simulink model "hydraulic_model"  (R2024a)
settings: Solver=ode23t  StartTime=0.0  StopTime=tEnd  FixedStep=1e-4  MaxStep=maxStep  RelTol=1e-2  AbsTol=1e-2
values from neighbouring files (symbols this model uses):
  boomHEArea = pi * (boomBoreDiameter/2)^2    (= 3117.24531052)    [init_model.m]
  boomREArea = pi * (boomBoreDiameter/2)^2 - pi*(boomRodDiameter/2)^2    (= 2410.38696347)    [init_model.m]
  swingDisplacement = 23.6    [init_model.m]
undefined symbols (not defined in the file or in its folder): ArmC, ArmR, AToTOrificeVector, BiPOrificeVector, BoomC, BoomR, boomValve, BToTOrificeVector, BucketC, BucketR, bucketValve, fluids, PToAOrificeVector, PToBOrificeVector, stickValve, SwingC, SwingR, swingValve, X, Y, Z
libraries: fl_lib x81, SimscapeFluids_lib x54, sm_lib x34, nesl_utility x29, spsFirstOrderFilterLib x4
(part 2 of 5)

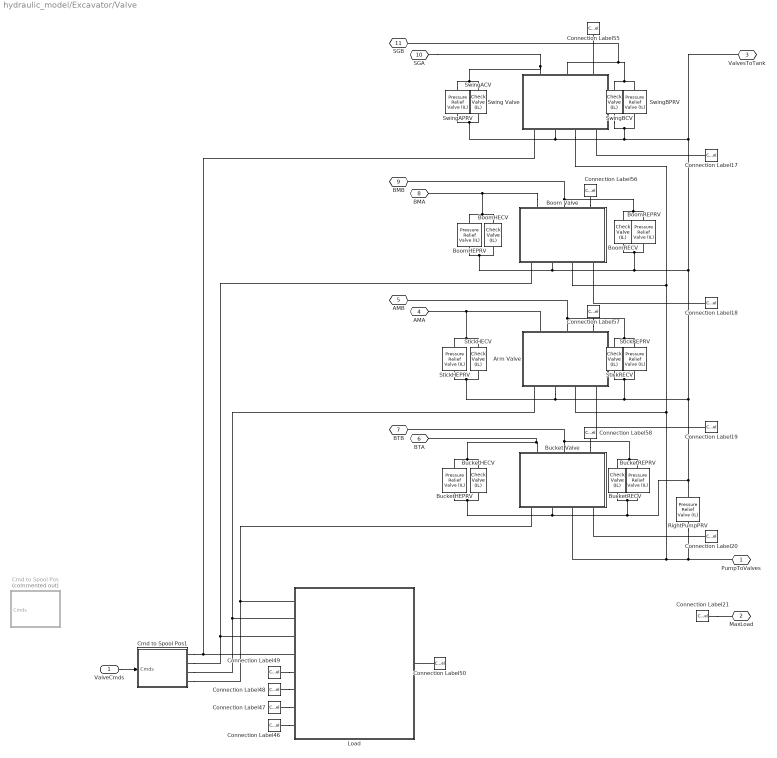
== system hydraulic_model/Excavator/Valve ==
  ValveCmds : Inport
  Arm Valve : Subsystem  mask{valveData=stickValve}
      mask prompts: valveData "Stick Valve Data Structure:"
      mask DialogControl DescGroupVar Prompt: Stick Valve
      mask DialogControl DescTextVar Prompt: The Stick Valve is a 6/3 valve with integrated check valve for induced flow.
      mask Display: image('Valve_6p3w_IMAGE.png');
  Boom Valve : Subsystem  mask{valveData=boomValve}
      mask prompts: valveData "Boom Valve Data Structure:"
      mask DialogControl DescGroupVar Prompt: Boom Valve
      mask DialogControl DescTextVar Prompt: The Boom Valve is a 6/3 valve with integrated check valve for induced flow.
      mask Display: image('Valve_6p3w_IMAGE.png');
  BoomHECV : SimscapeFluids_lib/Isothermal Liquid/Valves & Orifices/Directional Control Valves/Check Valve (IL)  opening_spec=2*(fluids.isothermal_liquid.valves_orifices.enum.opening_spec.linear)-1  pressure_control_spec=fluids.isothermal_liquid.valves_orifices.enum.pressure_control_spec.dp  p_crack_differential=checkValves.crackingPrDiff bar  p_crack_gauge=0.1 MPa  press_max_differential=checkValves.maxOpeningPrDiff bar  press_max_gauge=0.2 MPa  area_max=checkValves.maxOpeningArea mm^2  area_leak=checkValves.leakageArea mm^2  p_diff_TLU=[0.01 : 0.01 : 0.1] MPa  valve_area_TLU=[1e-10, 1e-05, 2e-05, 3e-05, 4e-05, 5e-05, 6e-05, 7.5e-05, 8.5e-05, .0001] m^2  vol_flow_TLU=[.000358, .045, .11, .191, .284, .39, .505, .63, .764, .905] .* 1e-3 m^3/s  area=inf m^2  Cd=0.64  Re_c=150  smoothing_factor=0.01  pressure_recovery=simscape.enum.onoff.off  opening_dynamics=simscape.enum.onoff.off  tau=0.1 s  enable_faults=simscape.enum.onoff.off  fault_action=fluids.enum.FaultOpening.Closed
      settings: InternalSimscapePortConfiguration="{\"Bottom\":[],\"Left\":[{\"id\":\"A\",\"label\":\"A\",\"type\":\"foundation.isothermal_liquid.isothermal_liquid\"}],\"Right\":[{\"id\":\"B\",\"label\":\"B\",\"type\":\"foundation.isothermal_liquid.isothermal_liquid\"}],\"Top\":[]}"
  BoomHEPRV : SimscapeFluids_lib/Isothermal Liquid/Valves & Orifices/Pressure Control Valves/Pressure Relief Valve (IL)  set_pressure_spec=foundation.enum.constant_controlled.constant  opening_spec=fluids.isothermal_liquid.valves_orifices.enum.opening_spec.linear  pressure_spec=fluids.isothermal_liquid.valves_orifices.enum.pressure_control_spec.dp  p_set_gauge=0.1 MPa  p_set_differential=fcnPRV.reliefPr bar  p_range=fcnPRV.regRange bar  area_max=fcnPRV.maxOpeningArea mm^2  area_leak=fcnPRV.leakageArea mm^2  p_diff_TLU=[0.2 : 0.2 : 1.2] MPa  p_gauge_TLU=[0.2 : 0.2 : 1.2] MPa  valve_area_TLU=[1e-10, 2e-06, 4e-06, 6e-06, 8e-06, 1e-05] m^2  vol_flow_TLU=[1e-09, 3.6e-05, 8.9e-05, .00015, .00023, .00031] m^3/s  area=inf m^2  Cd=0.64  Re_c=150  smoothing_factor=0.01  pressure_recovery=simscape.enum.onoff.off  opening_dynamics=simscape.enum.onoff.off  tau=0.1 s  enable_faults=simscape.enum.onoff.off  fault_type=fluids.enum.FaultOpening.Closed
      settings: InternalSimscapePortConfiguration="{\"Bottom\":[],\"Left\":[{\"id\":\"A\",\"label\":\"A\",\"type\":\"foundation.isothermal_liquid.isothermal_liquid\"}],\"Right\":[{\"id\":\"B\",\"label\":\"B\",\"type\":\"foundation.isothermal_liquid.isothermal_liquid\"}],\"Top\":[]}"
  BoomRECV : SimscapeFluids_lib/Isothermal Liquid/Valves & Orifices/Directional Control Valves/Check Valve (IL)  opening_spec=2*(fluids.isothermal_liquid.valves_orifices.enum.opening_spec.linear)-1  pressure_control_spec=fluids.isothermal_liquid.valves_orifices.enum.pressure_control_spec.dp  p_crack_differential=checkValves.crackingPrDiff bar  p_crack_gauge=0.1 MPa  press_max_differential=checkValves.maxOpeningPrDiff bar  press_max_gauge=0.2 MPa  area_max=checkValves.maxOpeningArea mm^2  area_leak=checkValves.leakageArea mm^2  p_diff_TLU=[0.01 : 0.01 : 0.1] MPa  valve_area_TLU=[1e-10, 1e-05, 2e-05, 3e-05, 4e-05, 5e-05, 6e-05, 7.5e-05, 8.5e-05, .0001] m^2  vol_flow_TLU=[.000358, .045, .11, .191, .284, .39, .505, .63, .764, .905] .* 1e-3 m^3/s  area=inf m^2  Cd=0.64  Re_c=150  smoothing_factor=0.01  pressure_recovery=simscape.enum.onoff.off  opening_dynamics=simscape.enum.onoff.off  tau=0.1 s  enable_faults=simscape.enum.onoff.off  fault_action=fluids.enum.FaultOpening.Closed
      settings: InternalSimscapePortConfiguration="{\"Bottom\":[],\"Left\":[{\"id\":\"A\",\"label\":\"A\",\"type\":\"foundation.isothermal_liquid.isothermal_liquid\"}],\"Right\":[{\"id\":\"B\",\"label\":\"B\",\"type\":\"foundation.isothermal_liquid.isothermal_liquid\"}],\"Top\":[]}"
  BoomREPRV : SimscapeFluids_lib/Isothermal Liquid/Valves & Orifices/Pressure Control Valves/Pressure Relief Valve (IL)  set_pressure_spec=foundation.enum.constant_controlled.constant  opening_spec=fluids.isothermal_liquid.valves_orifices.enum.opening_spec.linear  pressure_spec=fluids.isothermal_liquid.valves_orifices.enum.pressure_control_spec.dp  p_set_gauge=0.1 MPa  p_set_differential=fcnPRV.reliefPr bar  p_range=fcnPRV.regRange bar  area_max=fcnPRV.maxOpeningArea mm^2  area_leak=fcnPRV.leakageArea mm^2  p_diff_TLU=[0.2 : 0.2 : 1.2] MPa  p_gauge_TLU=[0.2 : 0.2 : 1.2] MPa  valve_area_TLU=[1e-10, 2e-06, 4e-06, 6e-06, 8e-06, 1e-05] m^2  vol_flow_TLU=[1e-09, 3.6e-05, 8.9e-05, .00015, .00023, .00031] m^3/s  area=inf m^2  Cd=0.64  Re_c=150  smoothing_factor=0.01  pressure_recovery=simscape.enum.onoff.off  opening_dynamics=simscape.enum.onoff.off  tau=0.1 s  enable_faults=simscape.enum.onoff.off  fault_type=fluids.enum.FaultOpening.Closed
      settings: InternalSimscapePortConfiguration="{\"Bottom\":[],\"Left\":[{\"id\":\"A\",\"label\":\"A\",\"type\":\"foundation.isothermal_liquid.isothermal_liquid\"}],\"Right\":[{\"id\":\"B\",\"label\":\"B\",\"type\":\"foundation.isothermal_liquid.isothermal_liquid\"}],\"Top\":[]}"
  Bucket Valve : Subsystem  mask{valveData=bucketValve}
      mask prompts: valveData "Bucket Valve Data Structure:"
      mask DialogControl DescGroupVar Prompt: Bucket Valve
      mask DialogControl DescTextVar Prompt: The Bucket Valve is a 6/3 valve.
      mask Display: image('Valve_6p3w_IMAGE.png');
  BucketHECV : SimscapeFluids_lib/Isothermal Liquid/Valves & Orifices/Directional Control Valves/Check Valve (IL)  opening_spec=2*(fluids.isothermal_liquid.valves_orifices.enum.opening_spec.linear)-1  pressure_control_spec=fluids.isothermal_liquid.valves_orifices.enum.pressure_control_spec.dp  p_crack_differential=checkValves.crackingPrDiff bar  p_crack_gauge=0.1 MPa  press_max_differential=checkValves.maxOpeningPrDiff bar  press_max_gauge=0.2 MPa  area_max=checkValves.maxOpeningArea mm^2  area_leak=checkValves.leakageArea mm^2  p_diff_TLU=[0.01 : 0.01 : 0.1] MPa  valve_area_TLU=[1e-10, 1e-05, 2e-05, 3e-05, 4e-05, 5e-05, 6e-05, 7.5e-05, 8.5e-05, .0001] m^2  vol_flow_TLU=[.000358, .045, .11, .191, .284, .39, .505, .63, .764, .905] .* 1e-3 m^3/s  area=inf m^2  Cd=0.64  Re_c=150  smoothing_factor=0.01  pressure_recovery=simscape.enum.onoff.off  opening_dynamics=simscape.enum.onoff.off  tau=0.1 s  enable_faults=simscape.enum.onoff.off  fault_action=fluids.enum.FaultOpening.Closed
      settings: InternalSimscapePortConfiguration="{\"Bottom\":[],\"Left\":[{\"id\":\"A\",\"label\":\"A\",\"type\":\"foundation.isothermal_liquid.isothermal_liquid\"}],\"Right\":[{\"id\":\"B\",\"label\":\"B\",\"type\":\"foundation.isothermal_liquid.isothermal_liquid\"}],\"Top\":[]}"
  BucketHEPRV : SimscapeFluids_lib/Isothermal Liquid/Valves & Orifices/Pressure Control Valves/Pressure Relief Valve (IL)  set_pressure_spec=foundation.enum.constant_controlled.constant  opening_spec=fluids.isothermal_liquid.valves_orifices.enum.opening_spec.linear  pressure_spec=fluids.isothermal_liquid.valves_orifices.enum.pressure_control_spec.dp  p_set_gauge=0.1 MPa  p_set_differential=fcnPRV.reliefPr bar  p_range=fcnPRV.regRange bar  area_max=fcnPRV.maxOpeningArea mm^2  area_leak=fcnPRV.leakageArea mm^2  p_diff_TLU=[0.2 : 0.2 : 1.2] MPa  p_gauge_TLU=[0.2 : 0.2 : 1.2] MPa  valve_area_TLU=[1e-10, 2e-06, 4e-06, 6e-06, 8e-06, 1e-05] m^2  vol_flow_TLU=[1e-09, 3.6e-05, 8.9e-05, .00015, .00023, .00031] m^3/s  area=inf m^2  Cd=0.64  Re_c=150  smoothing_factor=0.01  pressure_recovery=simscape.enum.onoff.off  opening_dynamics=simscape.enum.onoff.off  tau=0.1 s  enable_faults=simscape.enum.onoff.off  fault_type=fluids.enum.FaultOpening.Closed
      settings: InternalSimscapePortConfiguration="{\"Bottom\":[],\"Left\":[{\"id\":\"A\",\"label\":\"A\",\"type\":\"foundation.isothermal_liquid.isothermal_liquid\"}],\"Right\":[{\"id\":\"B\",\"label\":\"B\",\"type\":\"foundation.isothermal_liquid.isothermal_liquid\"}],\"Top\":[]}"
  BucketRECV : SimscapeFluids_lib/Isothermal Liquid/Valves & Orifices/Directional Control Valves/Check Valve (IL)  opening_spec=2*(fluids.isothermal_liquid.valves_orifices.enum.opening_spec.linear)-1  pressure_control_spec=fluids.isothermal_liquid.valves_orifices.enum.pressure_control_spec.dp  p_crack_differential=checkValves.crackingPrDiff bar  p_crack_gauge=0.1 MPa  press_max_differential=checkValves.maxOpeningPrDiff bar  press_max_gauge=0.2 MPa  area_max=checkValves.maxOpeningArea mm^2  area_leak=checkValves.leakageArea mm^2  p_diff_TLU=[0.01 : 0.01 : 0.1] MPa  valve_area_TLU=[1e-10, 1e-05, 2e-05, 3e-05, 4e-05, 5e-05, 6e-05, 7.5e-05, 8.5e-05, .0001] m^2  vol_flow_TLU=[.000358, .045, .11, .191, .284, .39, .505, .63, .764, .905] .* 1e-3 m^3/s  area=inf m^2  Cd=0.64  Re_c=150  smoothing_factor=0.01  pressure_recovery=simscape.enum.onoff.off  opening_dynamics=simscape.enum.onoff.off  tau=0.1 s  enable_faults=simscape.enum.onoff.off  fault_action=fluids.enum.FaultOpening.Closed
      settings: InternalSimscapePortConfiguration="{\"Bottom\":[],\"Left\":[{\"id\":\"A\",\"label\":\"A\",\"type\":\"foundation.isothermal_liquid.isothermal_liquid\"}],\"Right\":[{\"id\":\"B\",\"label\":\"B\",\"type\":\"foundation.isothermal_liquid.isothermal_liquid\"}],\"Top\":[]}"
  BucketREPRV : SimscapeFluids_lib/Isothermal Liquid/Valves & Orifices/Pressure Control Valves/Pressure Relief Valve (IL)  set_pressure_spec=foundation.enum.constant_controlled.constant  opening_spec=fluids.isothermal_liquid.valves_orifices.enum.opening_spec.linear  pressure_spec=fluids.isothermal_liquid.valves_orifices.enum.pressure_control_spec.dp  p_set_gauge=0.1 MPa  p_set_differential=fcnPRV.reliefPr bar  p_range=fcnPRV.regRange bar  area_max=fcnPRV.maxOpeningArea mm^2  area_leak=fcnPRV.leakageArea mm^2  p_diff_TLU=[0.2 : 0.2 : 1.2] MPa  p_gauge_TLU=[0.2 : 0.2 : 1.2] MPa  valve_area_TLU=[1e-10, 2e-06, 4e-06, 6e-06, 8e-06, 1e-05] m^2  vol_flow_TLU=[1e-09, 3.6e-05, 8.9e-05, .00015, .00023, .00031] m^3/s  area=inf m^2  Cd=0.64  Re_c=150  smoothing_factor=0.01  pressure_recovery=simscape.enum.onoff.off  opening_dynamics=simscape.enum.onoff.off  tau=0.1 s  enable_faults=simscape.enum.onoff.off  fault_type=fluids.enum.FaultOpening.Closed
      settings: InternalSimscapePortConfiguration="{\"Bottom\":[],\"Left\":[{\"id\":\"A\",\"label\":\"A\",\"type\":\"foundation.isothermal_liquid.isothermal_liquid\"}],\"Right\":[{\"id\":\"B\",\"label\":\"B\",\"type\":\"foundation.isothermal_liquid.isothermal_liquid\"}],\"Top\":[]}"
  Cmd to Spool Pos : Subsystem  Commented=on
  Cmd to Spool Pos1 : Subsystem
  Connection Label{17..21,50} (6 alike) : ConnectionLabel  Label=MaxLoad
  Connection Label46 : ConnectionLabel  Label=LoadSG
  Connection Label47 : ConnectionLabel  Label=LoadBM
  Connection Label48 : ConnectionLabel  Label=LoadAM
  Connection Label49 : ConnectionLabel  Label=LoadBT
  Connection Label55 : ConnectionLabel  Label=LoadSG
  Connection Label56 : ConnectionLabel  Label=LoadBM
  Connection Label57 : ConnectionLabel  Label=LoadAM
  Connection Label58 : ConnectionLabel  Label=LoadBT
  Load : Subsystem
  RightPumpPRV : SimscapeFluids_lib/Isothermal Liquid/Valves & Orifices/Pressure Control Valves/Pressure Relief Valve (IL)  set_pressure_spec=foundation.enum.constant_controlled.constant  opening_spec=fluids.isothermal_liquid.valves_orifices.enum.opening_spec.linear  pressure_spec=fluids.isothermal_liquid.valves_orifices.enum.pressure_control_spec.dp  p_set_gauge=0.1 MPa  p_set_differential=pumpPRV.reliefPr bar  p_range=pumpPRV.regRange bar  area_max=pumpPRV.maxOpeningArea mm^2  area_leak=pumpPRV.leakageArea mm^2  p_diff_TLU=[30.15e5 : 15e3 : 31.35e5] Pa  p_gauge_TLU=[30.15e5 : 15e3 : 31.35e5] Pa  valve_area_TLU=[1 : 1 : 9] .* 1e-5 m^2  vol_flow_TLU=[1e-09, 3.6e-05, 8.9e-05, .00015, .00023, .00031] m^3/s  area=inf m^2  Cd=0.64  Re_c=150  smoothing_factor=0.1  pressure_recovery=simscape.enum.onoff.off  opening_dynamics=simscape.enum.onoff.off  tau=0.1 s  enable_faults=simscape.enum.onoff.off  fault_type=fluids.enum.FaultOpening.Closed
      settings: InternalSimscapePortConfiguration="{\"Bottom\":[],\"Left\":[{\"id\":\"A\",\"label\":\"A\",\"type\":\"foundation.isothermal_liquid.isothermal_liquid\"}],\"Right\":[{\"id\":\"B\",\"label\":\"B\",\"type\":\"foundation.isothermal_liquid.isothermal_liquid\"}],\"Top\":[]}"
  StickHECV : SimscapeFluids_lib/Isothermal Liquid/Valves & Orifices/Directional Control Valves/Check Valve (IL)  opening_spec=2*(fluids.isothermal_liquid.valves_orifices.enum.opening_spec.linear)-1  pressure_control_spec=fluids.isothermal_liquid.valves_orifices.enum.pressure_control_spec.dp  p_crack_differential=checkValves.crackingPrDiff bar  p_crack_gauge=0.1 MPa  press_max_differential=checkValves.maxOpeningPrDiff bar  press_max_gauge=0.2 MPa  area_max=checkValves.maxOpeningArea mm^2  area_leak=checkValves.leakageArea mm^2  p_diff_TLU=[0.01 : 0.01 : 0.1] MPa  valve_area_TLU=[1e-10, 1e-05, 2e-05, 3e-05, 4e-05, 5e-05, 6e-05, 7.5e-05, 8.5e-05, .0001] m^2  vol_flow_TLU=[.000358, .045, .11, .191, .284, .39, .505, .63, .764, .905] .* 1e-3 m^3/s  area=inf m^2  Cd=0.64  Re_c=150  smoothing_factor=0.01  pressure_recovery=simscape.enum.onoff.off  opening_dynamics=simscape.enum.onoff.off  tau=0.1 s  enable_faults=simscape.enum.onoff.off  fault_action=fluids.enum.FaultOpening.Closed
      settings: InternalSimscapePortConfiguration="{\"Bottom\":[],\"Left\":[{\"id\":\"A\",\"label\":\"A\",\"type\":\"foundation.isothermal_liquid.isothermal_liquid\"}],\"Right\":[{\"id\":\"B\",\"label\":\"B\",\"type\":\"foundation.isothermal_liquid.isothermal_liquid\"}],\"Top\":[]}"
  StickHEPRV : SimscapeFluids_lib/Isothermal Liquid/Valves & Orifices/Pressure Control Valves/Pressure Relief Valve (IL)  set_pressure_spec=foundation.enum.constant_controlled.constant  opening_spec=fluids.isothermal_liquid.valves_orifices.enum.opening_spec.linear  pressure_spec=fluids.isothermal_liquid.valves_orifices.enum.pressure_control_spec.dp  p_set_gauge=0.1 MPa  p_set_differential=fcnPRV.reliefPr bar  p_range=fcnPRV.regRange bar  area_max=fcnPRV.maxOpeningArea mm^2  area_leak=fcnPRV.leakageArea mm^2  p_diff_TLU=[0.2 : 0.2 : 1.2] MPa  p_gauge_TLU=[0.2 : 0.2 : 1.2] MPa  valve_area_TLU=[1e-10, 2e-06, 4e-06, 6e-06, 8e-06, 1e-05] m^2  vol_flow_TLU=[1e-09, 3.6e-05, 8.9e-05, .00015, .00023, .00031] m^3/s  area=inf m^2  Cd=0.64  Re_c=150  smoothing_factor=0.01  pressure_recovery=simscape.enum.onoff.off  opening_dynamics=simscape.enum.onoff.off  tau=0.1 s  enable_faults=simscape.enum.onoff.off  fault_type=fluids.enum.FaultOpening.Closed
      settings: InternalSimscapePortConfiguration="{\"Bottom\":[],\"Left\":[{\"id\":\"A\",\"label\":\"A\",\"type\":\"foundation.isothermal_liquid.isothermal_liquid\"}],\"Right\":[{\"id\":\"B\",\"label\":\"B\",\"type\":\"foundation.isothermal_liquid.isothermal_liquid\"}],\"Top\":[]}"
  StickRECV : SimscapeFluids_lib/Isothermal Liquid/Valves & Orifices/Directional Control Valves/Check Valve (IL)  opening_spec=2*(fluids.isothermal_liquid.valves_orifices.enum.opening_spec.linear)-1  pressure_control_spec=fluids.isothermal_liquid.valves_orifices.enum.pressure_control_spec.dp  p_crack_differential=checkValves.crackingPrDiff bar  p_crack_gauge=0.1 MPa  press_max_differential=checkValves.maxOpeningPrDiff bar  press_max_gauge=0.2 MPa  area_max=checkValves.maxOpeningArea mm^2  area_leak=checkValves.leakageArea mm^2  p_diff_TLU=[0.01 : 0.01 : 0.1] MPa  valve_area_TLU=[1e-10, 1e-05, 2e-05, 3e-05, 4e-05, 5e-05, 6e-05, 7.5e-05, 8.5e-05, .0001] m^2  vol_flow_TLU=[.000358, .045, .11, .191, .284, .39, .505, .63, .764, .905] .* 1e-3 m^3/s  area=inf m^2  Cd=0.64  Re_c=150  smoothing_factor=0.01  pressure_recovery=simscape.enum.onoff.off  opening_dynamics=simscape.enum.onoff.off  tau=0.1 s  enable_faults=simscape.enum.onoff.off  fault_action=fluids.enum.FaultOpening.Closed
      settings: InternalSimscapePortConfiguration="{\"Bottom\":[],\"Left\":[{\"id\":\"A\",\"label\":\"A\",\"type\":\"foundation.isothermal_liquid.isothermal_liquid\"}],\"Right\":[{\"id\":\"B\",\"label\":\"B\",\"type\":\"foundation.isothermal_liquid.isothermal_liquid\"}],\"Top\":[]}"
  StickREPRV : SimscapeFluids_lib/Isothermal Liquid/Valves & Orifices/Pressure Control Valves/Pressure Relief Valve (IL)  set_pressure_spec=foundation.enum.constant_controlled.constant  opening_spec=fluids.isothermal_liquid.valves_orifices.enum.opening_spec.linear  pressure_spec=fluids.isothermal_liquid.valves_orifices.enum.pressure_control_spec.dp  p_set_gauge=0.1 MPa  p_set_differential=fcnPRV.reliefPr bar  p_range=fcnPRV.regRange bar  area_max=fcnPRV.maxOpeningArea mm^2  area_leak=fcnPRV.leakageArea mm^2  p_diff_TLU=[0.2 : 0.2 : 1.2] MPa  p_gauge_TLU=[0.2 : 0.2 : 1.2] MPa  valve_area_TLU=[1e-10, 2e-06, 4e-06, 6e-06, 8e-06, 1e-05] m^2  vol_flow_TLU=[1e-09, 3.6e-05, 8.9e-05, .00015, .00023, .00031] m^3/s  area=inf m^2  Cd=0.64  Re_c=150  smoothing_factor=0.01  pressure_recovery=simscape.enum.onoff.off  opening_dynamics=simscape.enum.onoff.off  tau=0.1 s  enable_faults=simscape.enum.onoff.off  fault_type=fluids.enum.FaultOpening.Closed
      settings: InternalSimscapePortConfiguration="{\"Bottom\":[],\"Left\":[{\"id\":\"A\",\"label\":\"A\",\"type\":\"foundation.isothermal_liquid.isothermal_liquid\"}],\"Right\":[{\"id\":\"B\",\"label\":\"B\",\"type\":\"foundation.isothermal_liquid.isothermal_liquid\"}],\"Top\":[]}"
  Swing Valve : Subsystem  mask{valveData=swingValve}
      mask prompts: valveData "Swing Valve Data Structure:"
      mask DialogControl DescGroupVar Prompt: Swing Valve
      mask DialogControl DescTextVar Prompt: The Swing Valve is a 6/3 valve.
      mask Display: image('Valve_6p3w_IMAGE.png');
  SwingACV : SimscapeFluids_lib/Isothermal Liquid/Valves & Orifices/Directional Control Valves/Check Valve (IL)  opening_spec=2*(fluids.isothermal_liquid.valves_orifices.enum.opening_spec.linear)-1  pressure_control_spec=fluids.isothermal_liquid.valves_orifices.enum.pressure_control_spec.dp  p_crack_differential=checkValves.crackingPrDiff bar  p_crack_gauge=0.1 MPa  press_max_differential=checkValves.maxOpeningPrDiff bar  press_max_gauge=0.2 MPa  area_max=checkValves.maxOpeningArea mm^2  area_leak=checkValves.leakageArea mm^2  p_diff_TLU=[0.01 : 0.01 : 0.1] MPa  valve_area_TLU=[1e-10, 1e-05, 2e-05, 3e-05, 4e-05, 5e-05, 6e-05, 7.5e-05, 8.5e-05, .0001] m^2  vol_flow_TLU=[.000358, .045, .11, .191, .284, .39, .505, .63, .764, .905] .* 1e-3 m^3/s  area=inf m^2  Cd=0.64  Re_c=150  smoothing_factor=0.01  pressure_recovery=simscape.enum.onoff.off  opening_dynamics=simscape.enum.onoff.off  tau=0.1 s  enable_faults=simscape.enum.onoff.off  fault_action=fluids.enum.FaultOpening.Closed
      settings: InternalSimscapePortConfiguration="{\"Bottom\":[],\"Left\":[{\"id\":\"A\",\"label\":\"A\",\"type\":\"foundation.isothermal_liquid.isothermal_liquid\"}],\"Right\":[{\"id\":\"B\",\"label\":\"B\",\"type\":\"foundation.isothermal_liquid.isothermal_liquid\"}],\"Top\":[]}"
  SwingAPRV : SimscapeFluids_lib/Isothermal Liquid/Valves & Orifices/Pressure Control Valves/Pressure Relief Valve (IL)  set_pressure_spec=foundation.enum.constant_controlled.constant  opening_spec=fluids.isothermal_liquid.valves_orifices.enum.opening_spec.linear  pressure_spec=fluids.isothermal_liquid.valves_orifices.enum.pressure_control_spec.dp  p_set_gauge=0.1 MPa  p_set_differential=swingPRV.reliefPr bar  p_range=swingPRV.regRange bar  area_max=swingPRV.maxOpeningArea mm^2  area_leak=swingPRV.leakageArea mm^2  p_diff_TLU=[0.2 : 0.2 : 1.2] MPa  p_gauge_TLU=[0.2 : 0.2 : 1.2] MPa  valve_area_TLU=[1e-10, 2e-06, 4e-06, 6e-06, 8e-06, 1e-05] m^2  vol_flow_TLU=[1e-09, 3.6e-05, 8.9e-05, .00015, .00023, .00031] m^3/s  area=inf m^2  Cd=0.64  Re_c=150  smoothing_factor=0.01  pressure_recovery=simscape.enum.onoff.off  opening_dynamics=simscape.enum.onoff.off  tau=0.1 s  enable_faults=simscape.enum.onoff.off  fault_type=fluids.enum.FaultOpening.Closed
      settings: InternalSimscapePortConfiguration="{\"Bottom\":[],\"Left\":[{\"id\":\"A\",\"label\":\"A\",\"type\":\"foundation.isothermal_liquid.isothermal_liquid\"}],\"Right\":[{\"id\":\"B\",\"label\":\"B\",\"type\":\"foundation.isothermal_liquid.isothermal_liquid\"}],\"Top\":[]}"
  SwingBCV : SimscapeFluids_lib/Isothermal Liquid/Valves & Orifices/Directional Control Valves/Check Valve (IL)  opening_spec=2*(fluids.isothermal_liquid.valves_orifices.enum.opening_spec.linear)-1  pressure_control_spec=fluids.isothermal_liquid.valves_orifices.enum.pressure_control_spec.dp  p_crack_differential=checkValves.crackingPrDiff bar  p_crack_gauge=0.1 MPa  press_max_differential=checkValves.maxOpeningPrDiff bar  press_max_gauge=0.2 MPa  area_max=checkValves.maxOpeningArea mm^2  area_leak=checkValves.leakageArea mm^2  p_diff_TLU=[0.01 : 0.01 : 0.1] MPa  valve_area_TLU=[1e-10, 1e-05, 2e-05, 3e-05, 4e-05, 5e-05, 6e-05, 7.5e-05, 8.5e-05, .0001] m^2  vol_flow_TLU=[.000358, .045, .11, .191, .284, .39, .505, .63, .764, .905] .* 1e-3 m^3/s  area=inf m^2  Cd=0.64  Re_c=150  smoothing_factor=0.01  pressure_recovery=simscape.enum.onoff.off  opening_dynamics=simscape.enum.onoff.off  tau=0.1 s  enable_faults=simscape.enum.onoff.off  fault_action=fluids.enum.FaultOpening.Closed
      settings: InternalSimscapePortConfiguration="{\"Bottom\":[],\"Left\":[{\"id\":\"A\",\"label\":\"A\",\"type\":\"foundation.isothermal_liquid.isothermal_liquid\"}],\"Right\":[{\"id\":\"B\",\"label\":\"B\",\"type\":\"foundation.isothermal_liquid.isothermal_liquid\"}],\"Top\":[]}"
  SwingBPRV : SimscapeFluids_lib/Isothermal Liquid/Valves & Orifices/Pressure Control Valves/Pressure Relief Valve (IL)  set_pressure_spec=foundation.enum.constant_controlled.constant  opening_spec=fluids.isothermal_liquid.valves_orifices.enum.opening_spec.linear  pressure_spec=fluids.isothermal_liquid.valves_orifices.enum.pressure_control_spec.dp  p_set_gauge=0.1 MPa  p_set_differential=swingPRV.reliefPr bar  p_range=swingPRV.regRange bar  area_max=swingPRV.maxOpeningArea mm^2  area_leak=swingPRV.leakageArea mm^2  p_diff_TLU=[0.2 : 0.2 : 1.2] MPa  p_gauge_TLU=[0.2 : 0.2 : 1.2] MPa  valve_area_TLU=[1e-10, 2e-06, 4e-06, 6e-06, 8e-06, 1e-05] m^2  vol_flow_TLU=[1e-09, 3.6e-05, 8.9e-05, .00015, .00023, .00031] m^3/s  area=inf m^2  Cd=0.64  Re_c=150  smoothing_factor=0.01  pressure_recovery=simscape.enum.onoff.off  opening_dynamics=simscape.enum.onoff.off  tau=0.1 s  enable_faults=simscape.enum.onoff.off  fault_type=fluids.enum.FaultOpening.Closed
      settings: InternalSimscapePortConfiguration="{\"Bottom\":[],\"Left\":[{\"id\":\"A\",\"label\":\"A\",\"type\":\"foundation.isothermal_liquid.isothermal_liquid\"}],\"Right\":[{\"id\":\"B\",\"label\":\"B\",\"type\":\"foundation.isothermal_liquid.isothermal_liquid\"}],\"Top\":[]}"
  PumpToValves : PMIOPort  Side=Left
  MaxLoad : PMIOPort  Port=2  Side=Left
  ValvesToTank : PMIOPort  Port=3  Side=Left
  AMA : PMIOPort  Port=4  Side=Right
  AMB : PMIOPort  Port=5  Side=Right
  BTA : PMIOPort  Port=6  Side=Right
  BTB : PMIOPort  Port=7  Side=Right
  BMA : PMIOPort  Port=8  Side=Right
  BMB : PMIOPort  Port=9  Side=Right
  SGA : PMIOPort  Port=10  Side=Right
  SGB : PMIOPort  Port=11  Side=Right
  wires:
  ValveCmds/1 -> Cmd to Spool Pos1/1(Cmds)
  connections:
  AMA/RConn1 -- StickHECV/RConn1 -- StickHEPRV/LConn1 -- Arm Valve/RConn1
  SwingBPRV/LConn1 -- SwingBCV/RConn1 -- SGB/RConn1 -- Swing Valve/RConn2
  BTA/RConn1 -- Bucket Valve/RConn1 -- BucketHECV/RConn1 -- BucketHEPRV/LConn1
  Bucket Valve/RConn2 -- BucketRECV/RConn1 -- BucketREPRV/LConn1 -- BTB/RConn1
  StickREPRV/LConn1 -- StickRECV/RConn1 -- Arm Valve/RConn2 -- AMB/RConn1
  SwingAPRV/LConn1 -- SGA/RConn1 -- Swing Valve/RConn1 -- SwingACV/RConn1
  Connection Label17/LConn1 -- Swing Valve/LConn4
  Connection Label19/LConn1 -- Arm Valve/LConn4
  Connection Label20/LConn1 -- Bucket Valve/LConn4
  Connection Label21/LConn1 -- MaxLoad/RConn1
  Connection Label18/LConn1 -- Boom Valve/LConn4
  SwingBPRV/RConn1 -- Swing Valve/LConn2 -- SwingACV/LConn1 -- SwingAPRV/RConn1 -- ValvesToTank/RConn1 -- BucketHEPRV/RConn1 -- BucketHECV/LConn1 -- Bucket Valve/LConn2 -- BucketREPRV/RConn1 -- BucketRECV/LConn1 -- RightPumpPRV/RConn1 -- StickHECV/LConn1 -- StickHEPRV/RConn1 -- Arm Valve/LConn2 -- StickRECV/LConn1 -- StickREPRV/RConn1 -- BoomHEPRV/RConn1 -- BoomHECV/LConn1 -- Boom Valve/LConn2 -- BoomRECV/LConn1 -- BoomREPRV/RConn1 -- SwingBCV/LConn1
  Swing Valve/LConn3 -- Boom Valve/LConn3 -- Arm Valve/LConn3 -- Bucket Valve/LConn3 -- PumpToValves/RConn1 -- RightPumpPRV/LConn1
  Connection Label55/LConn1 -- Swing Valve/RConn3
  Connection Label56/LConn1 -- Boom Valve/RConn3
  Connection Label57/LConn1 -- Arm Valve/RConn3
  Connection Label58/LConn1 -- Bucket Valve/RConn3
  Connection Label46/LConn1 -- Load/LConn8
  Connection Label47/LConn1 -- Load/LConn7
  Connection Label48/LConn1 -- Load/LConn6
  Connection Label49/LConn1 -- Load/LConn5
  Connection Label50/LConn1 -- Load/RConn1
  Boom Valve/RConn2 -- BoomREPRV/LConn1 -- BoomRECV/RConn1 -- BMB/RConn1
  Boom Valve/RConn1 -- BMA/RConn1 -- BoomHEPRV/LConn1 -- BoomHECV/RConn1
  Cmd to Spool Pos1/RConn1 -- Load/LConn4 -- Swing Valve/LConn1
  Cmd to Spool Pos1/RConn2 -- Load/LConn3 -- Boom Valve/LConn1
  Cmd to Spool Pos1/RConn3 -- Load/LConn2 -- Arm Valve/LConn1
  Cmd to Spool Pos1/RConn4 -- Load/LConn1 -- Bucket Valve/LConn1

== system hydraulic_model/Excavator/Functions/Arm ==
  ArmCylinder : SimscapeFluids_lib/Isothermal Liquid/Actuators/Double-Acting Actuator (IL)  single_fluid=true  mech_orientation=foundation.enum.MechOrientationTranslational.Positive  piston_area_A=stickHEArea mm^2  piston_area_B=stickREArea mm^2  stroke=stickStroke mm  dead_volume_A=1e-3 m^3  dead_volume_B=1e-3 m^3  pressure_spec=foundation.enum.pressure_spec.atmospheric  environment_pressure=0.101325 MPa  hardstop_model=simscape.enum.hardstop.smooth  stiff_coeff=1e8 N/m  damping_coeff=1e5 N/(m/s)  transition=0.1 mm  coeff_rest=0.7  v_tol=0.001 m/s  f_tol=0.001 N  cushion_A_spec=simscape.enum.onoff.off  area_plunger_A=1e-4 m^2  length_plunger_A=1e-3 m  area_cushion_orifice_A=1e-6 m^2  area_leak_plunger_A=1e-7 m^2  p_crack_differential_A=0.01 MPa  press_max_differential_A=0.1 MPa  check_valve_area_max_A=1e-4 m^2  check_valve_area_leak_A=1e-10 m^2  smoothing_factor_A=0  cushion_B_spec=simscape.enum.onoff.off  area_plunger_B=1e-4 m^2  length_plunger_B=1e-3 m  area_cushion_orifice_B=1e-6 m^2  area_leak_plunger_B=1e-7 m^2  p_crack_differential_B=0.01 MPa  press_max_differential_B=0.1 MPa  check_valve_area_max_B=1e-4 m^2  check_valve_area_leak_B=1e-10 m^2  smoothing_factor_B=0  friction_spec=true  breakaway_Coulomb_ratio=stickCylFriction.brkawyToCoulRatio  breakaway_velocity=stickCylFriction.brkawyVel m/s  preload_force=stickCylFriction.preloadForce N  Coulomb_coeff=stickCylFriction.coulForceCoef N/Pa  viscous_coeff=stickCylFriction.viscCoeff N/(m/s)  leakage_spec=simscape.enum.onoff.off  clearance=1e-4 m  piston_length=0.01 m  displacement_spec=foundation.enum.DisplacementSpec.Calculate  x0=initStickPistonPos m  dynamic_compressibility=simscape.enum.onoff.on  p0_A=initStickHEPr bar  p0_B=initStickREPr bar
      settings: InternalSimscapePortConfiguration="{\"Bottom\":[],\"Left\":[{\"id\":\"C\",\"label\":\"C\",\"type\":\"foundation.mechanical.translational.translational\"},{\"id\":\"A\",\"label\":\"A\",\"type\":\"foundation.isothermal_liquid.isothermal_liquid\"}],\"Right\":[{\"id\":\"p_out\",\"label\":\"p\",\"type\":\"output\"},{\"id\":\"R\",\"label\":\"R\",\"type\":\"foundation.mechanical.translational.translational\"},{\"id\":\"B\",\"label\":\"B\",\"type\":\"foundation.isothermal_liquid.isothermal_liquid\"}],\"Top\":[]}"
  BoomTranslationalRef1 : fl_lib/Mechanical/Translational Elements/Mechanical Translational Reference
  Ideal Translational Motion Sensor : fl_lib/Mechanical/Mechanical Sensors/Ideal Translational Motion Sensor  reference=foundation.enum.MeasurementReference.difference  acceleration_port=false  velocity_port=true  position_port=true  offset=armBias m
  PS Terminator : fl_lib/Physical Signals/Sinks/PS Terminator
  PS-Simulink Converter3 : nesl_utility/PS-Simulink Converter  PhysicalDomain=network_engine_domain  SubClassName=ps_output  LeftPortType=input  RightPortType=output  PseudoPeriodic=off  Frequencies=[]  VectorFormat=1-D array  Unit=m  AffineConversion=off
  PS-Simulink Converter5 : nesl_utility/PS-Simulink Converter  PhysicalDomain=network_engine_domain  SubClassName=ps_output  LeftPortType=input  RightPortType=output  PseudoPeriodic=off  Frequencies=[]  VectorFormat=1-D array  Unit=m/s  AffineConversion=off
  Simscape Bus : SimscapeBus  HierarchyStrings=ArmC;ArmR
  StickTranslationalRef : fl_lib/Mechanical/Translational Elements/Mechanical Translational Reference
  To Workspace : ToWorkspace  VariableName=posArm  SampleTime=-1
      settings: Save2DSignal=2-D array (concatenate along first dimension)
  To Workspace2 : ToWorkspace  VariableName=velArm  SampleTime=-1
      settings: Save2DSignal=2-D array (concatenate along first dimension)
  ArmA : PMIOPort  Side=Left
  ArmB : PMIOPort  Port=2  Side=Left
  ArmHydToMech : PMIOPort  Port=3  Side=Right
  wires:
  PS-Simulink Converter5/1 -> To Workspace2/1
  PS-Simulink Converter3/1 -> To Workspace/1
  connections:
  Ideal Translational Motion Sensor/LConn1 -- ArmCylinder/RConn2 -- Simscape Bus/LConn2
  ArmCylinder/RConn3 -- ArmB/RConn1
  ArmCylinder/LConn2 -- ArmA/RConn1
  ArmCylinder/LConn1 -- Simscape Bus/LConn1 -- StickTranslationalRef/LConn1
  BoomTranslationalRef1/LConn1 -- Ideal Translational Motion Sensor/RConn1
  PS-Simulink Converter3/LConn1 -- Ideal Translational Motion Sensor/RConn3
  Simscape Bus/RConn1 -- ArmHydToMech/RConn1
  PS-Simulink Converter5/LConn1 -- Ideal Translational Motion Sensor/RConn2
  ArmCylinder/RConn1 -- PS Terminator/LConn1

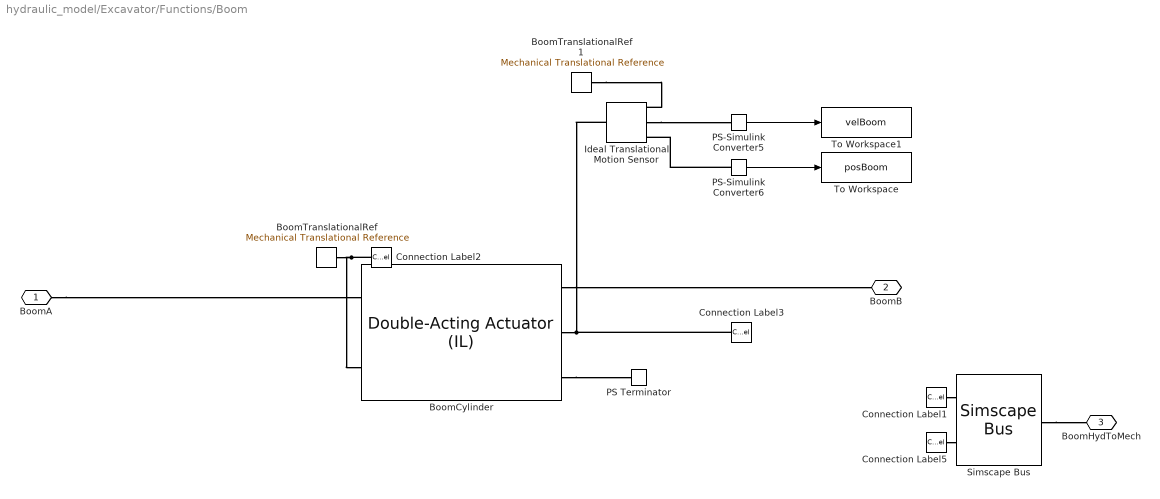
== system hydraulic_model/Excavator/Functions/Boom ==
  BoomCylinder : SimscapeFluids_lib/Isothermal Liquid/Actuators/Double-Acting Actuator (IL)  single_fluid=true  mech_orientation=foundation.enum.MechOrientationTranslational.Positive  piston_area_A=boomHEArea mm^2  piston_area_B=boomREArea mm^2  stroke=boomStroke mm  dead_volume_A=1e-4 m^3  dead_volume_B=1e-4 m^3  pressure_spec=foundation.enum.pressure_spec.atmospheric  environment_pressure=0.101325 MPa  hardstop_model=simscape.enum.hardstop.smooth  stiff_coeff=1e8 N/m  damping_coeff=1e5 N/(m/s)  transition=0.1 mm  coeff_rest=0.7  v_tol=0.001 m/s  f_tol=0.001 N  cushion_A_spec=false  area_plunger_A=boomHEArea/3 mm^2  length_plunger_A=5 mm  area_cushion_orifice_A=5 mm^2  area_leak_plunger_A=1e-7 m^2  p_crack_differential_A=0.01 MPa  press_max_differential_A=0.1 MPa  check_valve_area_max_A=1e-4 m^2  check_valve_area_leak_A=1e-10 m^2  smoothing_factor_A=0  cushion_B_spec=false  area_plunger_B=boomREArea/3 mm^2  length_plunger_B=5 mm  area_cushion_orifice_B=5 mm^2  area_leak_plunger_B=1e-7 m^2  p_crack_differential_B=0.01 MPa  press_max_differential_B=0.1 MPa  check_valve_area_max_B=1e-4 m^2  check_valve_area_leak_B=1e-10 m^2  smoothing_factor_B=0  friction_spec=true  breakaway_Coulomb_ratio=boomCylFriction.brkawyToCoulRatio  breakaway_velocity=boomCylFriction.brkawyVel m/s  preload_force=boomCylFriction.preloadForce N  Coulomb_coeff=boomCylFriction.coulForceCoef N/Pa  viscous_coeff=boomCylFriction.viscCoeff N/(m/s)  leakage_spec=simscape.enum.onoff.off  clearance=1e-4 m  piston_length=0.01 m  displacement_spec=foundation.enum.DisplacementSpec.Calculate  x0=initBoomPistonPos m  dynamic_compressibility=simscape.enum.onoff.on  p0_A=initBoomHEPr bar  p0_B=initBoomREPr bar
      settings: InternalSimscapePortConfiguration="{\"Bottom\":[],\"Left\":[{\"id\":\"C\",\"label\":\"C\",\"type\":\"foundation.mechanical.translational.translational\"},{\"id\":\"A\",\"label\":\"A\",\"type\":\"foundation.isothermal_liquid.isothermal_liquid\"}],\"Right\":[{\"id\":\"p_out\",\"label\":\"p\",\"type\":\"output\"},{\"id\":\"R\",\"label\":\"R\",\"type\":\"foundation.mechanical.translational.translational\"},{\"id\":\"B\",\"label\":\"B\",\"type\":\"foundation.isothermal_liquid.isothermal_liquid\"}],\"Top\":[]}"
  BoomTranslationalRef : fl_lib/Mechanical/Translational Elements/Mechanical Translational Reference
  BoomTranslationalRef1 : fl_lib/Mechanical/Translational Elements/Mechanical Translational Reference
  Connection Label1 : ConnectionLabel  Label=C
  Connection Label2 : ConnectionLabel  Label=C
  Connection Label3 : ConnectionLabel  Label=R
  Connection Label5 : ConnectionLabel  Label=R
  Ideal Translational Motion Sensor : fl_lib/Mechanical/Mechanical Sensors/Ideal Translational Motion Sensor  reference=foundation.enum.MeasurementReference.difference  acceleration_port=false  velocity_port=true  position_port=true  offset=boomBias m
  PS Terminator : fl_lib/Physical Signals/Sinks/PS Terminator
  PS-Simulink Converter5 : nesl_utility/PS-Simulink Converter  PhysicalDomain=network_engine_domain  SubClassName=ps_output  LeftPortType=input  RightPortType=output  PseudoPeriodic=off  Frequencies=[]  VectorFormat=1-D array  Unit=m/s  AffineConversion=off
  PS-Simulink Converter6 : nesl_utility/PS-Simulink Converter  PhysicalDomain=network_engine_domain  SubClassName=ps_output  LeftPortType=input  RightPortType=output  PseudoPeriodic=off  Frequencies=[]  VectorFormat=1-D array  Unit=m  AffineConversion=off
  Simscape Bus : SimscapeBus  HierarchyStrings=BoomC;BoomR
  To Workspace : ToWorkspace  VariableName=posBoom  SampleTime=-1
      settings: Save2DSignal=2-D array (concatenate along first dimension)
  To Workspace1 : ToWorkspace  VariableName=velBoom  SampleTime=-1
      settings: Save2DSignal=2-D array (concatenate along first dimension)
  BoomA : PMIOPort  Side=Left
  BoomB : PMIOPort  Port=2  Side=Left
  BoomHydToMech : PMIOPort  Port=3  Side=Right
  wires:
  PS-Simulink Converter5/1 -> To Workspace1/1
  PS-Simulink Converter6/1 -> To Workspace/1
  connections:
  BoomTranslationalRef/LConn1 -- BoomCylinder/LConn1 -- Connection Label2/LConn1
  BoomA/RConn1 -- BoomCylinder/LConn2
  BoomCylinder/RConn2 -- Connection Label3/LConn1 -- Ideal Translational Motion Sensor/LConn1
  BoomCylinder/RConn3 -- BoomB/RConn1
  BoomTranslationalRef1/LConn1 -- Ideal Translational Motion Sensor/RConn1
  Ideal Translational Motion Sensor/RConn2 -- PS-Simulink Converter5/LConn1
  PS-Simulink Converter6/LConn1 -- Ideal Translational Motion Sensor/RConn3
  Connection Label1/LConn1 -- Simscape Bus/LConn1
  Simscape Bus/RConn1 -- BoomHydToMech/RConn1
  Connection Label5/LConn1 -- Simscape Bus/LConn2
  BoomCylinder/RConn1 -- PS Terminator/LConn1

== system hydraulic_model/Excavator/Functions/Bucket ==
  BoomTranslationalRef1 : fl_lib/Mechanical/Translational Elements/Mechanical Translational Reference
  BucketCylinder : SimscapeFluids_lib/Isothermal Liquid/Actuators/Double-Acting Actuator (IL)  single_fluid=true  mech_orientation=foundation.enum.MechOrientationTranslational.Positive  piston_area_A=bucketHEArea mm^2  piston_area_B=bucketREArea mm^2  stroke=bucketStroke mm  dead_volume_A=5e-4 m^3  dead_volume_B=5e-4 m^3  pressure_spec=foundation.enum.pressure_spec.atmospheric  environment_pressure=0.101325 MPa  hardstop_model=simscape.enum.hardstop.smooth  stiff_coeff=1e8 N/m  damping_coeff=1e6 N/(m/s)  transition=0.1 mm  coeff_rest=0.7  v_tol=0.001 m/s  f_tol=0.001 N  cushion_A_spec=simscape.enum.onoff.off  area_plunger_A=1e-4 m^2  length_plunger_A=1e-3 m  area_cushion_orifice_A=1e-6 m^2  area_leak_plunger_A=1e-7 m^2  p_crack_differential_A=0.01 MPa  press_max_differential_A=0.1 MPa  check_valve_area_max_A=1e-4 m^2  check_valve_area_leak_A=1e-10 m^2  smoothing_factor_A=0  cushion_B_spec=simscape.enum.onoff.off  area_plunger_B=1e-4 m^2  length_plunger_B=1e-3 m  area_cushion_orifice_B=1e-6 m^2  area_leak_plunger_B=1e-7 m^2  p_crack_differential_B=0.01 MPa  press_max_differential_B=0.1 MPa  check_valve_area_max_B=1e-4 m^2  check_valve_area_leak_B=1e-10 m^2  smoothing_factor_B=0  friction_spec=true  breakaway_Coulomb_ratio=bucketCylFriction.brkawyToCoulRatio  breakaway_velocity=bucketCylFriction.brkawyVel m/s  preload_force=bucketCylFriction.preloadForce N  Coulomb_coeff=bucketCylFriction.coulForceCoef N/Pa  viscous_coeff=bucketCylFriction.viscCoeff N/(m/s)  leakage_spec=simscape.enum.onoff.off  clearance=1e-4 m  piston_length=0.01 m  displacement_spec=foundation.enum.DisplacementSpec.Calculate  x0=initBucketPistonPos m  dynamic_compressibility=simscape.enum.onoff.on  p0_A=initBucketHEPr bar  p0_B=initBucketREPr bar
      settings: InternalSimscapePortConfiguration="{\"Bottom\":[],\"Left\":[{\"id\":\"C\",\"label\":\"C\",\"type\":\"foundation.mechanical.translational.translational\"},{\"id\":\"A\",\"label\":\"A\",\"type\":\"foundation.isothermal_liquid.isothermal_liquid\"}],\"Right\":[{\"id\":\"p_out\",\"label\":\"p\",\"type\":\"output\"},{\"id\":\"R\",\"label\":\"R\",\"type\":\"foundation.mechanical.translational.translational\"},{\"id\":\"B\",\"label\":\"B\",\"type\":\"foundation.isothermal_liquid.isothermal_liquid\"}],\"Top\":[]}"
  BucketTranslationalRef : fl_lib/Mechanical/Translational Elements/Mechanical Translational Reference
  Ideal Translational Motion Sensor : fl_lib/Mechanical/Mechanical Sensors/Ideal Translational Motion Sensor  reference=foundation.enum.MeasurementReference.difference  acceleration_port=false  velocity_port=true  position_port=true  offset=bucketBias m
  PS Terminator : fl_lib/Physical Signals/Sinks/PS Terminator
  PS-Simulink Converter3 : nesl_utility/PS-Simulink Converter  PhysicalDomain=network_engine_domain  SubClassName=ps_output  LeftPortType=input  RightPortType=output  PseudoPeriodic=off  Frequencies=[]  VectorFormat=1-D array  Unit=m  AffineConversion=off
  PS-Simulink Converter5 : nesl_utility/PS-Simulink Converter  PhysicalDomain=network_engine_domain  SubClassName=ps_output  LeftPortType=input  RightPortType=output  PseudoPeriodic=off  Frequencies=[]  VectorFormat=1-D array  Unit=m/s  AffineConversion=off
  Simscape Bus : SimscapeBus  HierarchyStrings=BucketC;BucketR
  To Workspace2 : ToWorkspace  VariableName=posBucket  SampleTime=-1
      settings: Save2DSignal=2-D array (concatenate along first dimension)
  To Workspace3 : ToWorkspace  VariableName=velBucket  SampleTime=-1
      settings: Save2DSignal=2-D array (concatenate along first dimension)
  BucketA : PMIOPort  Side=Left
  BucketB : PMIOPort  Port=2  Side=Left
  BucketHydToMech : PMIOPort  Port=3  Side=Right
  wires:
  PS-Simulink Converter5/1 -> To Workspace3/1
  PS-Simulink Converter3/1 -> To Workspace2/1
  connections:
  Ideal Translational Motion Sensor/LConn1 -- Simscape Bus/LConn2 -- BucketCylinder/RConn2
  BucketCylinder/LConn2 -- BucketA/RConn1
  BucketTranslationalRef/LConn1 -- Simscape Bus/LConn1 -- BucketCylinder/LConn1
  BucketCylinder/RConn3 -- BucketB/RConn1
  BoomTranslationalRef1/LConn1 -- Ideal Translational Motion Sensor/RConn1
  Ideal Translational Motion Sensor/RConn2 -- PS-Simulink Converter5/LConn1
  PS-Simulink Converter3/LConn1 -- Ideal Translational Motion Sensor/RConn3
  Simscape Bus/RConn1 -- BucketHydToMech/RConn1
  BucketCylinder/RConn1 -- PS Terminator/LConn1

== system hydraulic_model/Excavator/Functions/Swing ==
  Motion Sensor : fl_lib/Mechanical/Mechanical Sensors/Ideal Rotational Motion Sensor  reference=foundation.enum.MeasurementReference.difference  acceleration_port=false  velocity_port=true  position_port=true  wrap_angle=false  offset=swingBias rad
  PS-Simulink Converter2 : nesl_utility/PS-Simulink Converter  PhysicalDomain=network_engine_domain  SubClassName=ps_output  LeftPortType=input  RightPortType=output  PseudoPeriodic=off  Frequencies=[]  VectorFormat=1-D array  Unit=rad  AffineConversion=off
  PS-Simulink Converter3 : nesl_utility/PS-Simulink Converter  PhysicalDomain=network_engine_domain  SubClassName=ps_output  LeftPortType=input  RightPortType=output  PseudoPeriodic=off  Frequencies=[]  VectorFormat=1-D array  Unit=rad/s  AffineConversion=off
  Simscape Bus : SimscapeBus  HierarchyStrings=SwingR;SwingC
  SwingGearBox : fl_lib/Mechanical/Mechanisms/Gear Box  ratio=swingGearRatio  t_in_specify=off  t_in_priority=None  t_in=0 N*m  t_in_nominal_specify=off  t_in_nominal_value=1  t_in_nominal_unit=N*m  t_out_specify=off  t_out_priority=None  t_out=0 N*m  t_out_nominal_specify=off  t_out_nominal_value=1  t_out_nominal_unit=N*m
  SwingMotor : SimscapeFluids_lib/Isothermal Liquid/Pumps & Motors/Fixed-Displacement Motor (IL)  leakage_friction_spec=fluids.isothermal_liquid.pumps_motors.enum.MotorLossSpec.Analytical  displacement=swingDisplacement cm^3/rev  omega_nominal=2000 rpm  p_nominal=216 bar  vol_eff_nominal=0.92  mech_eff_nominal=1 - (6283185.3072*(0.6e-6)/(swingDisplacement)) - (6283185.3072*(0.05)/(swingDisplacement)/(100e5))  no_load_torque=0.05 N*m  p_diff_eff_TLU=[100000, 1000000, 2000000] Pa  omega_eff_TLU=[25, 50, 100, 200, 300, 400] rad/s  vol_eff_TLU=[.816, .908, .954, .977, .981, .984; .325, .663, .831, .916, .925, .946; .137, .568, .78, .892, .893, .91]  mech_eff_TLU=[.996, .996, .996, .996, .996, .996; .988, .989, .989, .989, .989, .99; .981, .981, .982, .982, .983, .984]  p_diff_loss_TLU=[100000, 1000000, 2000000] Pa  omega_loss_TLU=[25, 50, 100, 200, 300, 400] rad/s  vol_loss_TLU=[.0282, .0253, .0241, .0235, .0291, .0325; .2596, .1271, .1017, .0917, .1216, .1142; .7874, .1901, .141, .1211, .1797, .1978] * 1e-3 m^3/s  mech_loss_TLU=[.002, .002, .002, .002, .002, .002; .06, .055, .055, .055, .055, .05; .19, .19, .18, .18, .17, .16] N*m  q_shaft_TLU=[.125, .25, .5, 1, 1.5, 2] * 1e-3 m^3/s  p_diff_shaft_TLU=[.1, 1, 2] MPa  torque_shaft_TLU=[.47, 4.72, 9.35; .47, 4.7, 9.36; .47, 4.7, 9.4; .47, 4.7, 9.41; .47, 4.7, 9.46; .47, 4.68, 9.5] N*m  omega_shaft_TLU=[205, 80, 35; 455, 330, 285; 955, 831, 780; 1950, 1830, 1780; 2940, 2775, 2680; 3940, 3780, 3640] rpm  vol_eff_min=1e-3  vol_eff_max=0.92  mech_eff_min=1e-3  mech_eff_max=0.88  pressure_threshold=1e5 Pa  omega_threshold=10 rad/s  supplied_range_check=simscape.enum.assert.action.none  motor_mode_check=simscape.enum.assert.action.none  pressure_check=simscape.enum.assert.action.none  p_min_valid=0 + 101325 Pa
      settings: InternalSimscapePortConfiguration="{\"Bottom\":[{\"id\":\"B\",\"label\":\"B\",\"type\":\"foundation.isothermal_liquid.isothermal_liquid\"}],\"Left\":[],\"Right\":[{\"id\":\"R\",\"label\":\"R\",\"type\":\"foundation.mechanical.rotational.rotational\"},{\"id\":\"C\",\"label\":\"C\",\"type\":\"foundation.mechanical.rotational.rotational\"}],\"Top\":[{\"id\":\"A\",\"label\":\"A\",\"type\":\"foundation.isothermal_liquid.isothermal_liquid\"}]}"
  SwingRotationalReference : fl_lib/Mechanical/Rotational Elements/Mechanical Rotational Reference
  To Workspace : ToWorkspace  VariableName=angSwing  SampleTime=-1
      settings: Save2DSignal=2-D array (concatenate along first dimension)
  To Workspace4 : ToWorkspace  VariableName=velSwing  SampleTime=-1
      settings: Save2DSignal=2-D array (concatenate along first dimension)
  SwingA : PMIOPort  Side=Left
  SwingB : PMIOPort  Port=2  Side=Left
  SwingHydToMech : PMIOPort  Port=3  Side=Right
  wires:
  PS-Simulink Converter2/1 -> To Workspace/1  "SwingAng"
  PS-Simulink Converter3/1 -> To Workspace4/1  "SwingVel"
  connections:
  SwingMotor/RConn1 -- SwingGearBox/LConn1
  SwingRotationalReference/LConn1 -- SwingMotor/RConn2 -- Simscape Bus/LConn2 -- Motion Sensor/RConn1
  Motion Sensor/LConn1 -- Simscape Bus/LConn1 -- SwingGearBox/RConn1
  SwingMotor/RConn3 -- SwingB/RConn1
  SwingA/RConn1 -- SwingMotor/LConn1
  PS-Simulink Converter2/LConn1 -- Motion Sensor/RConn3
  PS-Simulink Converter3/LConn1 -- Motion Sensor/RConn2
  SwingHydToMech/RConn1 -- Simscape Bus/RConn1
